simulink model "Signal"  (R2023a)
settings: Solver=VariableStepAuto  StartTime=0.0  StopTime=10.0  RelTol=1e-3
settings Model: Creator=paragmraw  LastModifiedBy=paragmraw

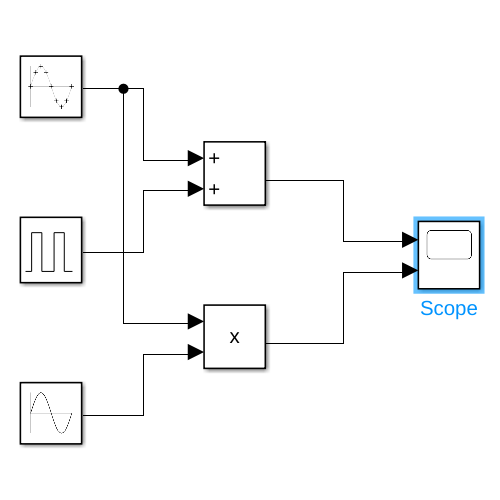
[thumbnail: Simulink's stored preview of the top-level diagram]
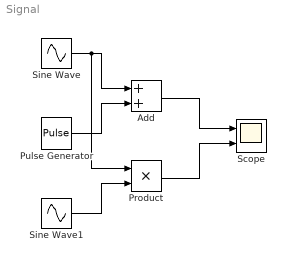
== system Signal ==
  Add : Sum
  Product : Product
  Pulse Generator : DiscretePulseGenerator  PulseType=Time based  Amplitude=10  Period=0.5  PulseWidth=50
  Scope : Scope  NumInputPorts=2
  Sine Wave : Sin  SineType=Sample based  Amplitude=10  Samples=50  SampleTime=0.5
  Sine Wave1 : Sin  Amplitude=10  Frequency=50  Samples=50  SampleTime=0
  wires:
  Sine Wave/1 -> Product/1, Add/1
  Pulse Generator/1 -> Add/2
  Sine Wave1/1 -> Product/2
  Add/1 -> Scope/1
  Product/1 -> Scope/2
